simulink model "Receive_Ethernet2024a_1"  (R2024a)
settings: Solver=FixedStepAuto  StartTime=0.0  StopTime=inf  FixedStep=0.01  RelTol=1e-3
undefined symbols (not defined in the file): gray
libraries: instrumentlib x2
settings Model: Creator=hyeon-yongjeong  LastModifiedBy=hyeon-yongjeong

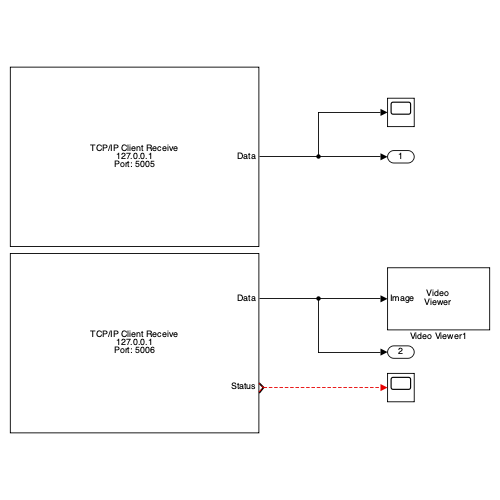
[thumbnail: Simulink's stored preview of the top-level diagram]
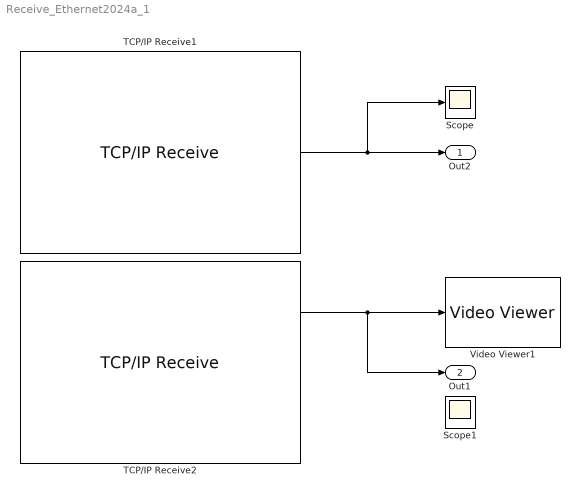
== system Receive_Ethernet2024a_1 ==
  Scope : Scope
  Scope1 : Scope
  TCP/IP Receive1 : instrumentlib/TCP//IP Receive  Host=127.0.0.1  Port=5005  DataSize=[ 7 1 ]  DataType=single  ASCIIFormatting=%f  Terminator=LF  CustomTerminator=10  ByteOrder=little-endian  EnableBlockingMode=on  Timeout=10  SampleTime=0.01  SimulateUsing=Interpreted execution
  TCP/IP Receive2 : instrumentlib/TCP//IP Receive  Host=127.0.0.1  Port=5006  DataSize=[240 320]  DataType=uint8  ASCIIFormatting=%f  Terminator=LF  CustomTerminator=10  ByteOrder=little-endian  EnableBlockingMode=off  Timeout=10  SampleTime=0.01  SimulateUsing=Interpreted execution
  Video Viewer1 : VideoViewer  colormapValue=gray(256)  FigPos=[815 770 636 450]
  Out2 : Outport
  Out1 : Outport  Port=2
  wires:
  TCP/IP Receive1/1 -> Scope/1, Out2/1
  TCP/IP Receive2/1 -> Out1/1, Video Viewer1/1
  ? -> Scope1/1
